simulink model "modelo_tanques_2_ordem"  (R2014a)
settings: Solver=ode3  StartTime=0.0  StopTime=100  FixedStep=0.1  RelTol=1e-3
settings Model: Creator=icaro  LastModifiedBy=Aluno IC

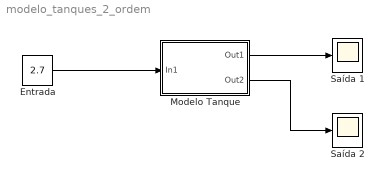
== system modelo_tanques_2_ordem ==
  Entrada : Constant  Value=2.7  SampleTime=.1
  Modelo Tanque : Subsystem
  Saída 1 : Scope
      settings: ShowLegends=on  TimeRange=100  YMin=0  YMax=30  SaveName=Saidajunta  SampleInput=on  SampleTime=10^-1
  Saída 2 : Scope
      settings: ShowLegends=on  TimeRange=100  YMin=0  YMax=30  SaveName=Saidajunta1  SampleInput=on  SampleTime=10^-1
  wires:
  Modelo Tanque/1(Out1) -> Saída 1/1
  Modelo Tanque/2(Out2) -> Saída 2/1
  Entrada/1 -> Modelo Tanque/1(In1)

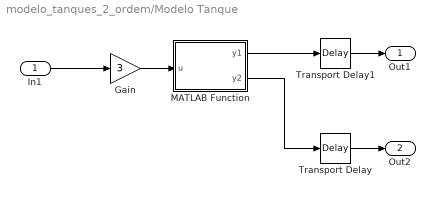
== system modelo_tanques_2_ordem/Modelo Tanque ==
  In1 : Inport
  Gain : Gain  Gain=3
  MATLAB Function : MATLAB Function  TreatAsAtomicUnit=on
  Transport Delay : TransportDelay  DelayTime=2
  Transport Delay1 : TransportDelay  DelayTime=2
  Out1 : Outport
  Out2 : Outport  Port=2
  wires:
  Gain/1 -> MATLAB Function/1(u)
  Transport Delay/1 -> Out2/1
  Transport Delay1/1 -> Out1/1
  MATLAB Function/1(y1) -> Transport Delay1/1
  MATLAB Function/2(y2) -> Transport Delay/1
  In1/1 -> Gain/1

== matlab function modelo_tanques_2_ordem/Modelo Tanque/MATLAB Function ==
  data: u input; y1 output; y2 output
function [y1, y2]= fcn(u)

persistent A1
persistent A2
persistent a1
persistent a2
persistent km
persistent g
persistent t
persistent h1
persistent h2

if(isempty(t))
    A1 = pi*(4.445/2)^2;           %Area transversal do tanque 1
    A2 = pi*(4.445/2)^2;           %Area transversal do tanque 2
    a1 = (0.445/2)^2*pi;     %Area transversal da tubulação de saida em t1 
    a2 =(0.445/2)^2*pi;    %Area transversal da tubulação de saida em t2
    km = 3.3;                %Constante do Motor
    g  = 980.665;               %Constante da gravidade
    h1 = 0;
    h2 = 0;
    t = 10^-1;
end

dh1 = ((km*u) - a1*sqrt(2*g*h1))/A1;
h1 = h1 + t*dh1;
if(h1<0)
    h1 = 0;
end
dh2 = (a1*sqrt(2*g*h1) - a2*sqrt(2*g*h2))/A2;
h2 = h2 + t*dh2;
if(h2<0)
    h2 = 0;
end

y1 = h1;
y2 = h2;

end
